simulink model "ricerca_errore_scalature"  (R2020b)
settings: Solver=VariableStepAuto  StartTime=0.0  StopTime=0.01  RelTol=1e-3
values from neighbouring files (symbols this model uses):
  attuatore_Amax = 20*(pi/180)    (= 0.349065850399)    [v2021_10_27_avvioSITL.m]    (also in v2021_10_27_calcoloAerodinamica.m)
  attuatore_Emax = 25*(pi/180)    (= 0.436332312999)    [v2021_10_27_avvioSITL.m]    (also in v2021_10_27_calcoloAerodinamica.m)
  attuatore_Rmax = 25*(pi/180)    (= 0.436332312999)    [v2021_10_27_avvioSITL.m]    (also in v2021_10_27_calcoloAerodinamica.m)
  deltaAtrim = 0    [v2021_10_27_avvioSITL.m]
  deltaEtrim = 0    [v2021_10_27_avvioSITL.m]
  deltaRtrim = 0    [v2021_10_27_avvioSITL.m]
  deltaTtrim = 0.1    [v2021_10_27_avvioSITL.m]
  PWM_Aileron = rad2deg(deltaAtrim)*9+1503    [v2021_10_27_avvioSITL.m]
  PWM_Elevator = rad2deg(deltaEtrim)*(447/50)+(3007/2)    [v2021_10_27_avvioSITL.m]
  PWM_Rudder = rad2deg(deltaRtrim)*(447/50)+(3007/2)    [v2021_10_27_avvioSITL.m]
  PWM_Throttle = (deltaTtrim)*800+1100    (= 1180)    [v2021_10_27_avvioSITL.m]
undefined symbols (not defined in the file or in its folder): State0
libraries: simulink_extras x24
settings Model: Creator=emanueledalessio  LastModifiedBy=emanueledalessio

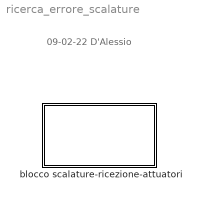
== system ricerca_errore_scalature ==
  note: 09-02-22 D'Alessio
  "blocco scalature-ricezione-attuatori " : Subsystem

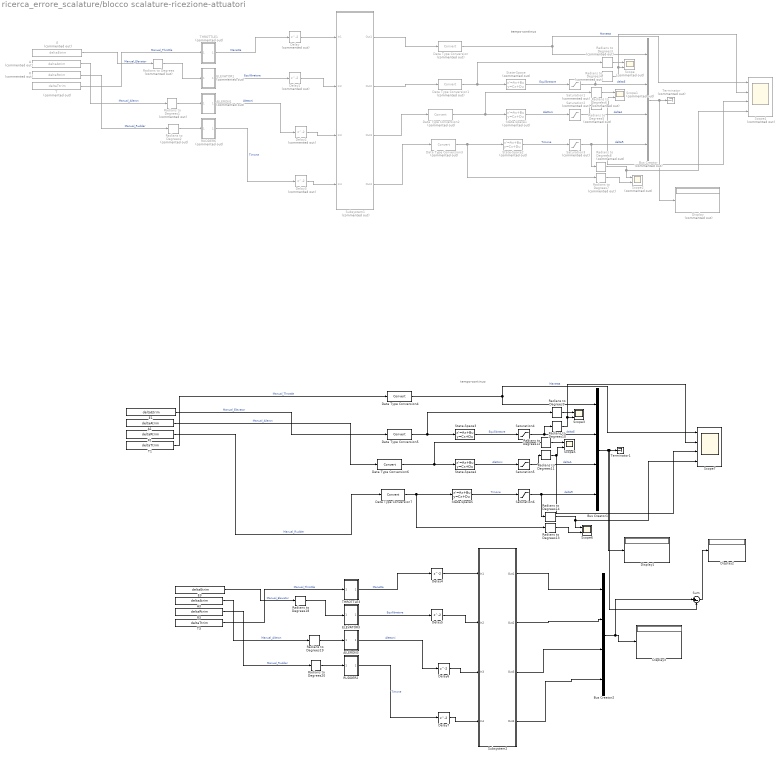
== system ricerca_errore_scalature/blocco scalature-ricezione-attuatori  ==
  note: tempo-continuo
  note: tempo-continuo
  A : Constant  Commented=on  Value=deltaAtrim  SampleTime=0.02
  A1 : Constant  Value=deltaAtrim  SampleTime=0.02
  A3 : Constant  Value=deltaAtrim  SampleTime=0.02
  AILERON1 : Subsystem  Commented=on
  AILERON3 : Subsystem
  Bus Creator : BusCreator  Commented=on  Inputs=4
  Bus Creator1 : BusCreator  Inputs=4
  Bus Creator2 : BusCreator  Inputs=4
  Data Type Conversion{,1..3} (4 alike) : DataTypeConversion  Commented=on
  Data Type Conversion{4..7} (4 alike) : DataTypeConversion
  Delay : Delay  Commented=on  InitialCondition=PWM_Throttle
  Delay1 : Delay  Commented=on  InitialCondition=PWM_Elevator
  Delay2 : Delay  Commented=on  InitialCondition=PWM_Aileron
  Delay3 : Delay  Commented=on  InitialCondition=PWM_Rudder
  Delay4 : Delay  InitialCondition=PWM_Throttle
  Delay5 : Delay  InitialCondition=PWM_Elevator
  Delay6 : Delay  InitialCondition=PWM_Aileron
  Delay7 : Delay  InitialCondition=PWM_Rudder
  Display : Display  Commented=on
  Display1 : Display
  Display2 : Display
  Display3 : Display
  E : Constant  Commented=on  Value=deltaEtrim  SampleTime=0.02
  E1 : Constant  Value=deltaEtrim  SampleTime=0.02
  E3 : Constant  Value=deltaEtrim  SampleTime=0.02
  ELEVATOR1 : Subsystem  Commented=on
  ELEVATOR3 : Subsystem
  R : Constant  Commented=on  Value=deltaRtrim  SampleTime=0.02
  R1 : Constant  Value=deltaRtrim  SampleTime=0.02
  R3 : Constant  Value=deltaRtrim  SampleTime=0.02
  RUDDER2 : Subsystem
  RUDDER6 : Subsystem  Commented=on
  Radians to Degrees{,1..8} (9 alike) : simulink_extras/Transformations/Radians to Degrees  Commented=on
  Radians to Degrees{9..14,18..20} (9 alike) : simulink_extras/Transformations/Radians to Degrees
  Saturation1 : Saturate  Commented=on  UpperLimit=attuatore_Emax+0.1  LowerLimit=-attuatore_Emax
  Saturation2 : Saturate  Commented=on  UpperLimit=attuatore_Amax+0.1  LowerLimit=-attuatore_Amax
  Saturation3 : Saturate  Commented=on  UpperLimit=attuatore_Rmax+0.1  LowerLimit=-attuatore_Rmax
  Saturation4 : Saturate  UpperLimit=attuatore_Emax+0.1  LowerLimit=-attuatore_Emax
  Saturation5 : Saturate  UpperLimit=attuatore_Amax+0.1  LowerLimit=-attuatore_Amax
  Saturation6 : Saturate  UpperLimit=attuatore_Rmax+0.1  LowerLimit=-attuatore_Rmax
  Scope : Scope  Commented=on  NumInputPorts=2
  Scope1 : Scope  Commented=on  NumInputPorts=2
  Scope2 : Scope  Commented=on  NumInputPorts=2
  Scope3 : Scope  NumInputPorts=2
  Scope4 : Scope  Commented=on  NumInputPorts=4
  Scope5 : Scope  NumInputPorts=2
  Scope6 : Scope  NumInputPorts=2
  Scope7 : Scope  NumInputPorts=4
  State-Space : StateSpace  Commented=on  A=-12.54  C=12.54  D=0  InitialCondition=State0.Ele0
  State-Space1 : StateSpace  Commented=on  A=-12.54  C=12.54  D=0  InitialCondition=State0.Ail0
  State-Space2 : StateSpace  Commented=on  A=-12.54  C=12.54  D=0  InitialCondition=State0.Rud0
  State-Space3 : StateSpace  A=-12.54  C=12.54  D=0  InitialCondition=State0.Ele0
  State-Space4 : StateSpace  A=-12.54  C=12.54  D=0  InitialCondition=State0.Ail0
  State-Space5 : StateSpace  A=-12.54  C=12.54  D=0  InitialCondition=State0.Rud0
  Subsystem1 : Subsystem  Commented=on  TreatAsAtomicUnit=on  SystemSampleTime=0.01
  Subsystem2 : Subsystem  TreatAsAtomicUnit=on  SystemSampleTime=0.01
  Sum : Sum  Inputs=|+-
  T : Constant  Commented=on  Value=deltaTtrim  SampleTime=0.02
  T1 : Constant  Value=deltaTtrim  SampleTime=0.02
  T3 : Constant  Value=deltaTtrim  SampleTime=0.02
  THROTTLE1 : Subsystem  Commented=on
  THROTTLE3 : Subsystem
  Terminator : Terminator  Commented=on
  Terminator1 : Terminator
  wires:
  ELEVATOR1/1(Out1) -> Delay1/1  "Equilibratore"
  RUDDER6/1(Out1) -> Delay3/1  "Timone"
  THROTTLE1/1(Out1) -> Delay/1  "Manetta"
  AILERON1/1(Out1) -> Delay2/1  "Alettoni"
  Radians to Degrees/1 -> ELEVATOR1/1(In1)
  Radians to Degrees1/1 -> AILERON1/1(In1)
  Radians to Degrees2/1 -> RUDDER6/1(In1)
  Delay2/1 -> Subsystem1/3(In3)
  Delay3/1 -> Subsystem1/4(In4)
  Delay1/1 -> Subsystem1/2(In2)
  Radians to Degrees8/1 -> Scope4/4, Scope2/1
  State-Space/1 -> Saturation1/1  "Equilibratore"
  Data Type Conversion1/1 -> State-Space/1, Radians to Degrees3/1
  Radians to Degrees3/1 -> Scope/1
  Radians to Degrees5/1 -> Scope4/3, Scope1/2
  State-Space2/1 -> Saturation3/1  "Timone"
  Saturation2/1 -> Radians to Degrees5/1, Bus Creator/3  "deltaA"
  Radians to Degrees6/1 -> Scope1/1
  Data Type Conversion/1 -> Bus Creator/1, Scope4/1  "Manetta"
  Bus Creator/1 -> Display/1, Terminator/1
  State-Space1/1 -> Saturation2/1  "Alettoni"
  Radians to Degrees4/1 -> Scope4/2, Scope/2
  Radians to Degrees7/1 -> Scope2/2
  Data Type Conversion3/1 -> State-Space2/1, Radians to Degrees7/1
  Saturation3/1 -> Radians to Degrees8/1, Bus Creator/4  "deltaR"
  Saturation1/1 -> Bus Creator/2, Radians to Degrees4/1  "deltaE"
  Data Type Conversion2/1 -> State-Space1/1, Radians to Degrees6/1
  E/1 -> Radians to Degrees/1  "Manual_Elevator"
  T/1 -> THROTTLE1/1(In1)  "Manual_Throttle"
  R/1 -> Radians to Degrees2/1  "Manual_Rudder"
  A/1 -> Radians to Degrees1/1  "Manual_Aileron"
  Subsystem1/1(Out1) -> Data Type Conversion/1
  Subsystem1/2(Out2) -> Data Type Conversion1/1
  Subsystem1/3(Out3) -> Data Type Conversion2/1
  Subsystem1/4(Out4) -> Data Type Conversion3/1
  Delay/1 -> Subsystem1/1(In1)
  Radians to Degrees12/1 -> Scope5/1
  Data Type Conversion5/1 -> State-Space3/1, Radians to Degrees9/1
  Radians to Degrees14/1 -> Scope7/4, Scope6/1
  Data Type Conversion4/1 -> Bus Creator1/1, Scope7/1  "Manetta"
  State-Space5/1 -> Saturation6/1  "Timone"
  Radians to Degrees10/1 -> Scope7/2, Scope3/2
  Radians to Degrees9/1 -> Scope3/1
  Saturation4/1 -> Bus Creator1/2, Radians to Degrees10/1  "deltaE"
  Radians to Degrees11/1 -> Scope7/3, Scope5/2
  Radians to Degrees13/1 -> Scope6/2
  Saturation6/1 -> Radians to Degrees14/1, Bus Creator1/4  "deltaR"
  Saturation5/1 -> Radians to Degrees11/1, Bus Creator1/3  "deltaA"
  Data Type Conversion6/1 -> State-Space4/1, Radians to Degrees12/1
  Bus Creator1/1 -> Terminator1/1, Sum/2, Display1/1
  State-Space4/1 -> Saturation5/1  "Alettoni"
  Data Type Conversion7/1 -> State-Space5/1, Radians to Degrees13/1
  State-Space3/1 -> Saturation4/1  "Equilibratore"
  E1/1 -> Data Type Conversion5/1  "Manual_Elevator"
  A1/1 -> Data Type Conversion6/1  "Manual_Aileron"
  T1/1 -> Data Type Conversion4/1  "Manual_Throttle"
  R1/1 -> Data Type Conversion7/1  "Manual_Rudder"
  Subsystem2/2(Out2) -> Bus Creator2/2
  AILERON3/1(Out1) -> Delay6/1  "Alettoni"
  THROTTLE3/1(Out1) -> Delay4/1  "Manetta"
  Subsystem2/1(Out1) -> Bus Creator2/1
  E3/1 -> Radians to Degrees18/1  "Manual_Elevator"
  Radians to Degrees20/1 -> RUDDER2/1(In1)
  Delay5/1 -> Subsystem2/2(In2)
  R3/1 -> Radians to Degrees20/1  "Manual_Rudder"
  Radians to Degrees18/1 -> ELEVATOR3/1(In1)
  A3/1 -> Radians to Degrees19/1  "Manual_Aileron"
  T3/1 -> THROTTLE3/1(In1)  "Manual_Throttle"
  RUDDER2/1(Out1) -> Delay7/1  "Timone"
  Delay7/1 -> Subsystem2/4(In4)
  ELEVATOR3/1(Out1) -> Delay5/1  "Equilibratore"
  Radians to Degrees19/1 -> AILERON3/1(In1)
  Subsystem2/4(Out4) -> Bus Creator2/4
  Delay4/1 -> Subsystem2/1(In1)
  Subsystem2/3(Out3) -> Bus Creator2/3
  Delay6/1 -> Subsystem2/3(In3)
  Bus Creator2/1 -> Sum/1, Display3/1
  Sum/1 -> Display2/1

== system ricerca_errore_scalature/blocco scalature-ricezione-attuatori /AILERON1 ==
  In1 : Inport
  Constant1 : Constant  Value=1503
  Gain : Gain  Gain=9
  Sum : Sum  Inputs=|++  OutDataTypeStr=int16
  Out1 : Outport  VectorParamsAs1DForOutWhenUnconnected=off
  wires:
  Gain/1 -> Sum/1
  Constant1/1 -> Sum/2
  In1/1 -> Gain/1
  Sum/1 -> Out1/1

== system ricerca_errore_scalature/blocco scalature-ricezione-attuatori /AILERON3 ==
  In1 : Inport
  Constant1 : Constant  Value=1503
  Gain : Gain  Gain=9
  Sum : Sum  Inputs=|++  OutDataTypeStr=int16
  Out1 : Outport  VectorParamsAs1DForOutWhenUnconnected=off
  wires:
  Gain/1 -> Sum/1
  Constant1/1 -> Sum/2
  In1/1 -> Gain/1
  Sum/1 -> Out1/1

== system ricerca_errore_scalature/blocco scalature-ricezione-attuatori /ELEVATOR1 ==
  In1 : Inport
  Constant1 : Constant  Value=3007/2
  Gain : Gain  Gain=447/50
  Sum : Sum  Inputs=|++  OutDataTypeStr=int16
  Out1 : Outport  VectorParamsAs1DForOutWhenUnconnected=off
  wires:
  Gain/1 -> Sum/1
  Constant1/1 -> Sum/2
  In1/1 -> Gain/1
  Sum/1 -> Out1/1

== system ricerca_errore_scalature/blocco scalature-ricezione-attuatori /ELEVATOR3 ==
  In1 : Inport
  Constant1 : Constant  Value=3007/2
  Gain : Gain  Gain=447/50
  Sum : Sum  Inputs=|++  OutDataTypeStr=int16
  Out1 : Outport  VectorParamsAs1DForOutWhenUnconnected=off
  wires:
  Gain/1 -> Sum/1
  Constant1/1 -> Sum/2
  In1/1 -> Gain/1
  Sum/1 -> Out1/1

== system ricerca_errore_scalature/blocco scalature-ricezione-attuatori /RUDDER2 ==
  In1 : Inport
  Constant1 : Constant  Value=3007/2
  Gain : Gain  Gain=447/50
  Sum : Sum  Inputs=|++  OutDataTypeStr=int16
  Out1 : Outport  VectorParamsAs1DForOutWhenUnconnected=off
  wires:
  Gain/1 -> Sum/1
  Constant1/1 -> Sum/2
  In1/1 -> Gain/1
  Sum/1 -> Out1/1

== system ricerca_errore_scalature/blocco scalature-ricezione-attuatori /RUDDER6 ==
  In1 : Inport
  Constant1 : Constant  Value=3007/2
  Gain : Gain  Gain=447/50
  Sum : Sum  Inputs=|++  OutDataTypeStr=int16
  Out1 : Outport  VectorParamsAs1DForOutWhenUnconnected=off
  wires:
  Gain/1 -> Sum/1
  Constant1/1 -> Sum/2
  In1/1 -> Gain/1
  Sum/1 -> Out1/1

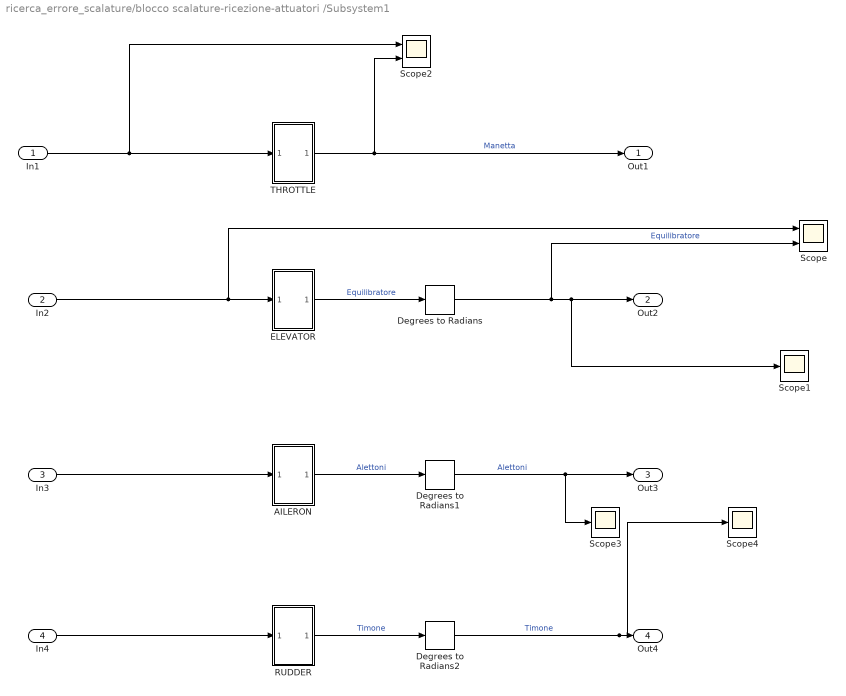
== system ricerca_errore_scalature/blocco scalature-ricezione-attuatori /Subsystem1 ==
  In1 : Inport
  In2 : Inport  Port=2
  In3 : Inport  Port=3
  In4 : Inport  Port=4
  AILERON : Subsystem
  Degrees to Radians : simulink_extras/Transformations/Degrees to Radians
  Degrees to Radians1 : simulink_extras/Transformations/Degrees to Radians
  Degrees to Radians2 : simulink_extras/Transformations/Degrees to Radians
  ELEVATOR : Subsystem
  RUDDER : Subsystem
  Scope : Scope  NumInputPorts=2
  Scope1 : Scope
  Scope2 : Scope  NumInputPorts=2
  Scope3 : Scope
  Scope4 : Scope
  THROTTLE : Subsystem
  Out1 : Outport  VectorParamsAs1DForOutWhenUnconnected=off
  Out2 : Outport  Port=2  VectorParamsAs1DForOutWhenUnconnected=off
  Out3 : Outport  Port=3  VectorParamsAs1DForOutWhenUnconnected=off
  Out4 : Outport  Port=4  VectorParamsAs1DForOutWhenUnconnected=off
  wires:
  In3/1 -> AILERON/1(In1)
  In4/1 -> RUDDER/1(In1)
  In2/1 -> Scope/1, ELEVATOR/1(In1)
  In1/1 -> Scope2/1, THROTTLE/1(In1)
  Degrees to Radians2/1 -> Out4/1, Scope4/1  "Timone"
  Degrees to Radians1/1 -> Out3/1, Scope3/1  "Alettoni"
  Degrees to Radians/1 -> Scope/2, Scope1/1, Out2/1  "Equilibratore"
  THROTTLE/1(Out1) -> Scope2/2, Out1/1  "Manetta"
  ELEVATOR/1(Out1) -> Degrees to Radians/1  "Equilibratore"
  AILERON/1(Out1) -> Degrees to Radians1/1  "Alettoni"
  RUDDER/1(Out1) -> Degrees to Radians2/1  "Timone"

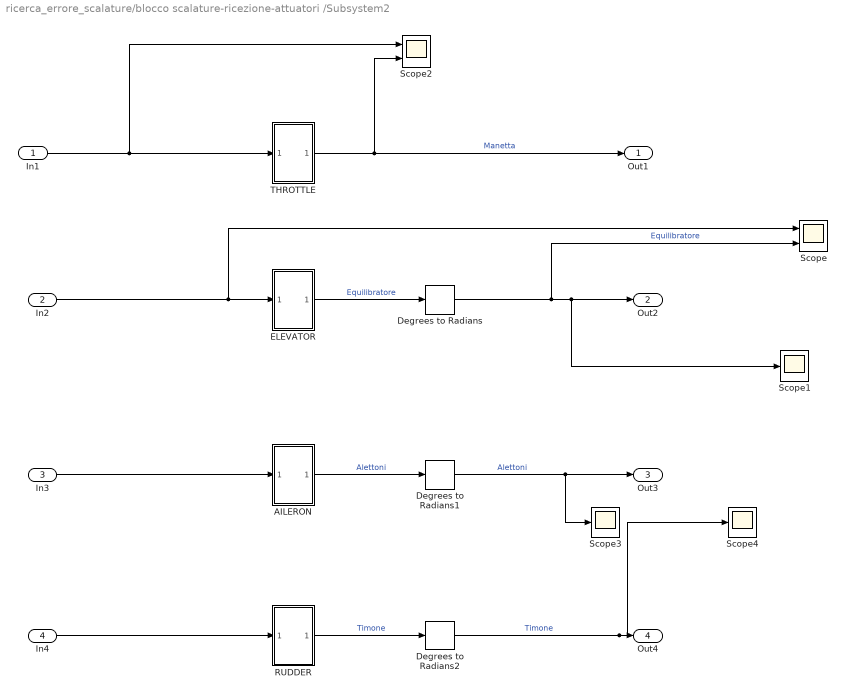
== system ricerca_errore_scalature/blocco scalature-ricezione-attuatori /Subsystem2 ==
  In1 : Inport
  In2 : Inport  Port=2
  In3 : Inport  Port=3
  In4 : Inport  Port=4
  AILERON : Subsystem
  Degrees to Radians : simulink_extras/Transformations/Degrees to Radians
  Degrees to Radians1 : simulink_extras/Transformations/Degrees to Radians
  Degrees to Radians2 : simulink_extras/Transformations/Degrees to Radians
  ELEVATOR : Subsystem
  RUDDER : Subsystem
  Scope : Scope  NumInputPorts=2
  Scope1 : Scope
  Scope2 : Scope  NumInputPorts=2
  Scope3 : Scope
  Scope4 : Scope
  THROTTLE : Subsystem
  Out1 : Outport  VectorParamsAs1DForOutWhenUnconnected=off
  Out2 : Outport  Port=2  VectorParamsAs1DForOutWhenUnconnected=off
  Out3 : Outport  Port=3  VectorParamsAs1DForOutWhenUnconnected=off
  Out4 : Outport  Port=4  VectorParamsAs1DForOutWhenUnconnected=off
  wires:
  In3/1 -> AILERON/1(In1)
  In4/1 -> RUDDER/1(In1)
  In2/1 -> Scope/1, ELEVATOR/1(In1)
  In1/1 -> Scope2/1, THROTTLE/1(In1)
  Degrees to Radians2/1 -> Out4/1, Scope4/1  "Timone"
  Degrees to Radians1/1 -> Out3/1, Scope3/1  "Alettoni"
  Degrees to Radians/1 -> Scope/2, Scope1/1, Out2/1  "Equilibratore"
  THROTTLE/1(Out1) -> Scope2/2, Out1/1  "Manetta"
  ELEVATOR/1(Out1) -> Degrees to Radians/1  "Equilibratore"
  AILERON/1(Out1) -> Degrees to Radians1/1  "Alettoni"
  RUDDER/1(Out1) -> Degrees to Radians2/1  "Timone"

== system ricerca_errore_scalature/blocco scalature-ricezione-attuatori /THROTTLE1 ==
  In1 : Inport
  Constant : Constant  Value=1100
  Gain : Gain  Gain=800
  Sum : Sum  Inputs=|++  AccumDataTypeStr=int16  OutDataTypeStr=int16
  Out1 : Outport  VectorParamsAs1DForOutWhenUnconnected=off
  wires:
  In1/1 -> Gain/1
  Gain/1 -> Sum/1
  Constant/1 -> Sum/2
  Sum/1 -> Out1/1

== system ricerca_errore_scalature/blocco scalature-ricezione-attuatori /THROTTLE3 ==
  In1 : Inport
  Constant : Constant  Value=1100
  Gain : Gain  Gain=800
  Sum : Sum  Inputs=|++  AccumDataTypeStr=int16  OutDataTypeStr=int16
  Out1 : Outport  VectorParamsAs1DForOutWhenUnconnected=off
  wires:
  In1/1 -> Gain/1
  Gain/1 -> Sum/1
  Constant/1 -> Sum/2
  Sum/1 -> Out1/1

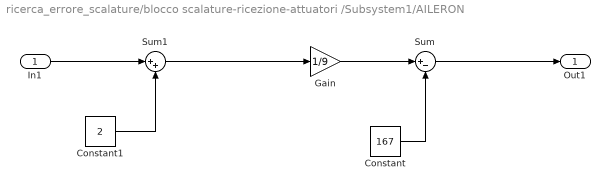
== system ricerca_errore_scalature/blocco scalature-ricezione-attuatori /Subsystem1/AILERON ==
  In1 : Inport
  Constant : Constant  Value=167
  Constant1 : Constant  Value=2
  Gain : Gain  Gain=1/9
  Sum : Sum  Inputs=|+-
  Sum1 : Sum  Inputs=|++
  Out1 : Outport  VectorParamsAs1DForOutWhenUnconnected=off
  wires:
  Gain/1 -> Sum/1
  Constant/1 -> Sum/2
  Sum/1 -> Out1/1
  In1/1 -> Sum1/1
  Sum1/1 -> Gain/1
  Constant1/1 -> Sum1/2

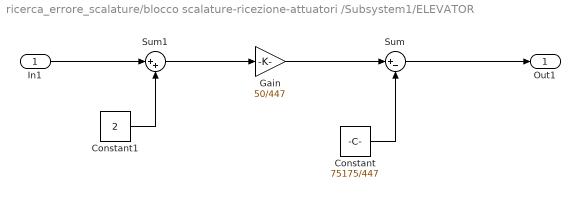
== system ricerca_errore_scalature/blocco scalature-ricezione-attuatori /Subsystem1/ELEVATOR ==
  In1 : Inport
  Constant : Constant  Value=75175/447
  Constant1 : Constant  Value=2
  Gain : Gain  Gain=50/447
  Sum : Sum  Inputs=|+-
  Sum1 : Sum  Inputs=|++
  Out1 : Outport  VectorParamsAs1DForOutWhenUnconnected=off
  wires:
  Sum1/1 -> Gain/1
  Constant/1 -> Sum/2
  Sum/1 -> Out1/1
  In1/1 -> Sum1/1
  Constant1/1 -> Sum1/2
  Gain/1 -> Sum/1

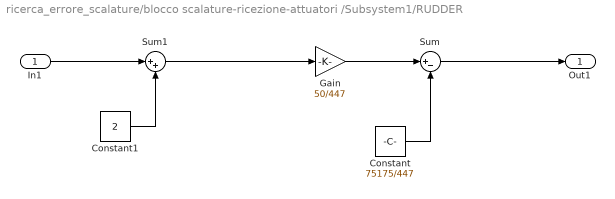
== system ricerca_errore_scalature/blocco scalature-ricezione-attuatori /Subsystem1/RUDDER ==
  In1 : Inport
  Constant : Constant  Value=75175/447
  Constant1 : Constant  Value=2
  Gain : Gain  Gain=50/447
  Sum : Sum  Inputs=|+-
  Sum1 : Sum  Inputs=|++
  Out1 : Outport  VectorParamsAs1DForOutWhenUnconnected=off
  wires:
  Gain/1 -> Sum/1
  Constant/1 -> Sum/2
  Sum/1 -> Out1/1
  In1/1 -> Sum1/1
  Sum1/1 -> Gain/1
  Constant1/1 -> Sum1/2

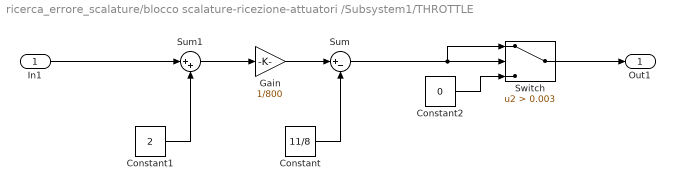
== system ricerca_errore_scalature/blocco scalature-ricezione-attuatori /Subsystem1/THROTTLE ==
  In1 : Inport
  Constant : Constant  Value=11/8
  Constant1 : Constant  Value=2
  Constant2 : Constant  Value=0
  Gain : Gain  Gain=1/800
  Sum : Sum  Inputs=|+-
  Sum1 : Sum  Inputs=|++
  Switch : Switch  Criteria=u2 > Threshold  Threshold=0.003
  Out1 : Outport  VectorParamsAs1DForOutWhenUnconnected=off
  wires:
  Sum1/1 -> Gain/1
  Constant/1 -> Sum/2
  In1/1 -> Sum1/1
  Constant1/1 -> Sum1/2
  Gain/1 -> Sum/1
  Switch/1 -> Out1/1
  Sum/1 -> Switch/1, Switch/2
  Constant2/1 -> Switch/3

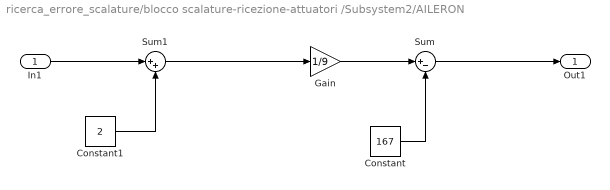
== system ricerca_errore_scalature/blocco scalature-ricezione-attuatori /Subsystem2/AILERON ==
  In1 : Inport
  Constant : Constant  Value=167
  Constant1 : Constant  Value=2
  Gain : Gain  Gain=1/9
  Sum : Sum  Inputs=|+-
  Sum1 : Sum  Inputs=|++
  Out1 : Outport  VectorParamsAs1DForOutWhenUnconnected=off
  wires:
  Gain/1 -> Sum/1
  Constant/1 -> Sum/2
  Sum/1 -> Out1/1
  In1/1 -> Sum1/1
  Sum1/1 -> Gain/1
  Constant1/1 -> Sum1/2

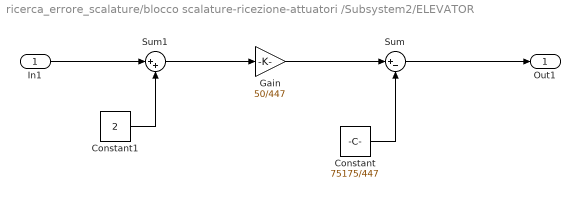
== system ricerca_errore_scalature/blocco scalature-ricezione-attuatori /Subsystem2/ELEVATOR ==
  In1 : Inport
  Constant : Constant  Value=75175/447
  Constant1 : Constant  Value=2
  Gain : Gain  Gain=50/447
  Sum : Sum  Inputs=|+-
  Sum1 : Sum  Inputs=|++
  Out1 : Outport  VectorParamsAs1DForOutWhenUnconnected=off
  wires:
  Sum1/1 -> Gain/1
  Constant/1 -> Sum/2
  Sum/1 -> Out1/1
  In1/1 -> Sum1/1
  Constant1/1 -> Sum1/2
  Gain/1 -> Sum/1

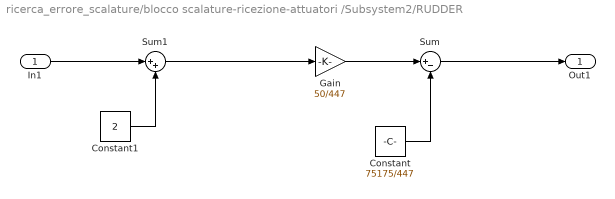
== system ricerca_errore_scalature/blocco scalature-ricezione-attuatori /Subsystem2/RUDDER ==
  In1 : Inport
  Constant : Constant  Value=75175/447
  Constant1 : Constant  Value=2
  Gain : Gain  Gain=50/447
  Sum : Sum  Inputs=|+-
  Sum1 : Sum  Inputs=|++
  Out1 : Outport  VectorParamsAs1DForOutWhenUnconnected=off
  wires:
  Gain/1 -> Sum/1
  Constant/1 -> Sum/2
  Sum/1 -> Out1/1
  In1/1 -> Sum1/1
  Sum1/1 -> Gain/1
  Constant1/1 -> Sum1/2

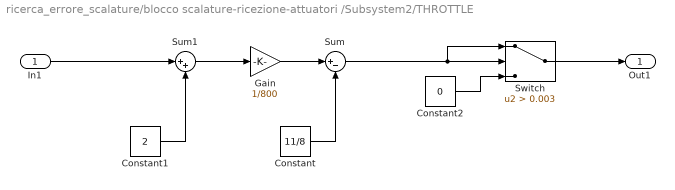
== system ricerca_errore_scalature/blocco scalature-ricezione-attuatori /Subsystem2/THROTTLE ==
  In1 : Inport
  Constant : Constant  Value=11/8
  Constant1 : Constant  Value=2
  Constant2 : Constant  Value=0
  Gain : Gain  Gain=1/800
  Sum : Sum  Inputs=|+-
  Sum1 : Sum  Inputs=|++
  Switch : Switch  Criteria=u2 > Threshold  Threshold=0.003
  Out1 : Outport  VectorParamsAs1DForOutWhenUnconnected=off
  wires:
  Sum1/1 -> Gain/1
  Constant/1 -> Sum/2
  In1/1 -> Sum1/1
  Constant1/1 -> Sum1/2
  Gain/1 -> Sum/1
  Switch/1 -> Out1/1
  Sum/1 -> Switch/1, Switch/2
  Constant2/1 -> Switch/3
